simulink model "simulink_2_7"  (R2018a)
settings: Solver=VariableStepAuto  StartTime=0.0  StopTime=20  RelTol=1e-3
settings Model: Creator=Ryan  LastModifiedBy=Ryan

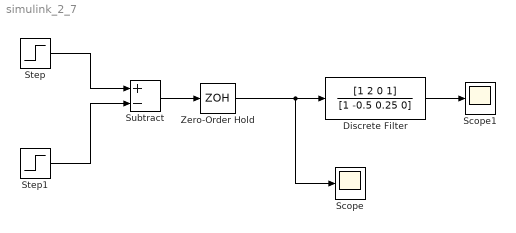
== system simulink_2_7 ==
  Discrete Filter : DiscreteFilter  Numerator=[1 2 0 1]  Denominator=[1 -0.5 0.25 0]
  Scope : Scope
  Scope1 : Scope
  Step : Step  Time=0  SampleTime=0
  Step1 : Step  SampleTime=0
  Subtract : Sum  Inputs=+-
  Zero-Order Hold : ZeroOrderHold
  wires:
  Step/1 -> Subtract/1
  Step1/1 -> Subtract/2
  Subtract/1 -> Zero-Order Hold/1
  Zero-Order Hold/1 -> Discrete Filter/1, Scope/1
  Discrete Filter/1 -> Scope1/1
